simulink model "rigidbodyA"  (Simulink 6.1)
settings: Solver=ode45  StartTime=0.0  StopTime=10.0  RelTol=1e-3
libraries: simulink x1
settings Model: LastModifiedBy=okawa
settings DebuggingCC: SolverPrmCheckMsg=warning

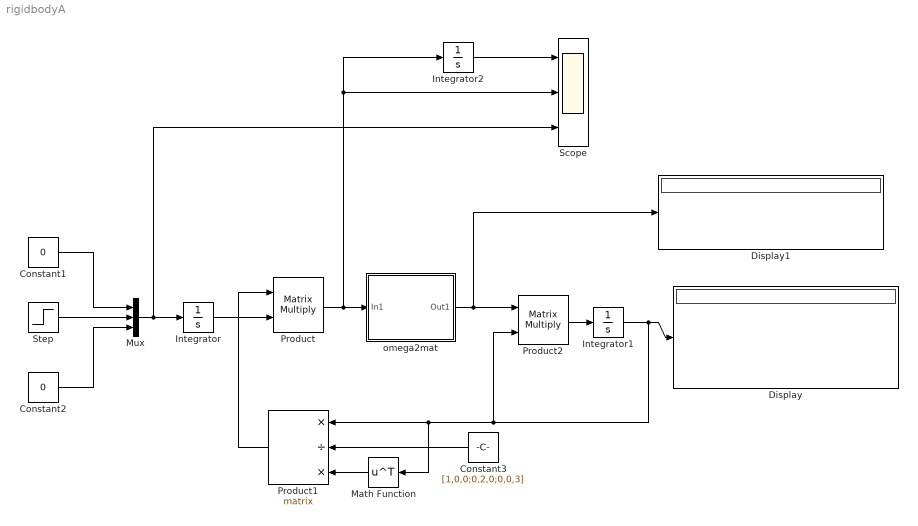
== system rigidbodyA ==
  Constant1 : Constant  Value=0
  Constant2 : Constant  Value=0
  Constant3 : Constant  Orientation=left  Value=[1,0,0;0,2,0;0,0,3]  VectorParams1D=off
  Display : Display
  Display1 : Display
  Integrator : Integrator
  Integrator1 : Integrator  InitialCondition=[1,0,0;0,1,0;0,0,1]
  Integrator2 : Integrator
  Math Function : Math  Orientation=left  Operator=transpose  SaturateOnIntegerOverflow=on
  Mux : Mux  Inputs=3
  Product : Product  Inputs=**  Multiplication=Matrix(*)  RndMeth=Zero
  Product1 : Product  Orientation=left  Inputs=*/*  Multiplication=Matrix(*)  RndMeth=Zero
  Product2 : Product  Inputs=**  Multiplication=Matrix(*)  RndMeth=Zero
  Scope : Scope  NumInputPorts=3
      settings: YMin=-5~-5~-5  YMax=5~5~5
  Step : Step  SampleTime=0
  omega2mat : Subsystem
  wires:
  Constant1/1 -> Mux/1
  Step/1 -> Mux/2
  Constant2/1 -> Mux/3
  Mux/1 -> Integrator/1, Scope/3
  Integrator/1 -> Product/2
  Product/1 -> omega2mat/1(In1), Scope/2, Integrator2/1
  omega2mat/1(Out1) -> Product2/1, Display1/1
  Product2/1 -> Integrator1/1
  Integrator1/1 -> Display/1, Product1/1, Math Function/1, Product2/2
  Constant3/1 -> Product1/2
  Math Function/1 -> Product1/3
  Integrator2/1 -> Scope/1
  Product1/1 -> Product/1

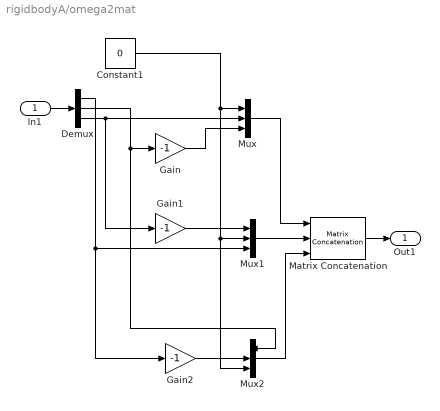
== system rigidbodyA/omega2mat ==
  In1 : Inport  Port=1  LatchInput=off
  Constant1 : Constant  Value=0
  Demux : Demux  Outputs=3
  Gain : Gain  Gain=-1
  Gain1 : Gain  Gain=-1
  Gain2 : Gain  Gain=-1
  Matrix Concatenation : simulink/Math Operations/Matrix Concatenation  numInports=3  catMethod=Horizontal
  Mux : Mux  Inputs=3
  Mux1 : Mux  Inputs=3
  Mux2 : Mux  Inputs=3
  Out1 : Outport
  wires:
  Constant1/1 -> Mux/1, Mux1/2, Mux2/3
  Demux/2 -> Gain/1, Mux2/1
  Gain/1 -> Mux/3
  Demux/3 -> Mux/2, Gain1/1
  Gain1/1 -> Mux1/1
  Demux/1 -> Mux1/3, Gain2/1
  Gain2/1 -> Mux2/2
  Mux/1 -> Matrix Concatenation/1
  Mux1/1 -> Matrix Concatenation/2
  Mux2/1 -> Matrix Concatenation/3
  In1/1 -> Demux/1
  Matrix Concatenation/1 -> Out1/1
